simulink model "sl_spmsm"  (R2023b)
settings: Solver=VariableStepAuto  StartTime=0.0  StopTime=10.0  RelTol=1e-3
InitFcn:
  | init
values from neighbouring files (symbols this model uses):
  pa = block.DialogPrm(1).Data    [SPMSM_abc_model.m]    (also in park.m; pwm.m; torque_equation.m; voltage_equation.m)
libraries: slpidlib x1
settings Model: Creator=PC  LastModifiedBy=PC

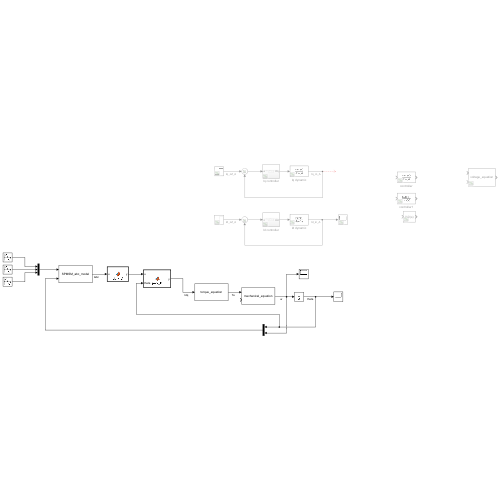
[thumbnail: Simulink's stored preview of the top-level diagram]
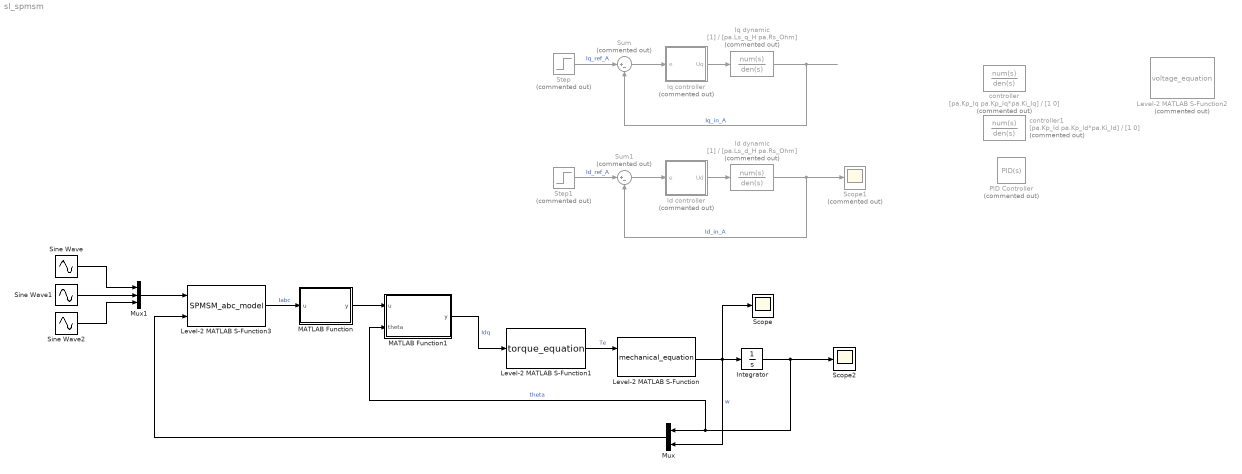
== system sl_spmsm ==
  Id controller : Subsystem  Commented=on
  Id dynamic : TransferFcn  Commented=on  Denominator=[pa.Ls_d_H pa.Rs_Ohm]
  Integrator : Integrator
  Iq controller : Subsystem  Commented=on
  Iq dynamic : TransferFcn  Commented=on  Denominator=[pa.Ls_q_H pa.Rs_Ohm]
  Level-2 MATLAB S-Function : M-S-Function  FunctionName=mechanical_equation  Parameters=pa
  Level-2 MATLAB S-Function1 : M-S-Function  FunctionName=torque_equation  Parameters=pa
  Level-2 MATLAB S-Function2 : M-S-Function  Commented=on  FunctionName=voltage_equation  Parameters=pa
  Level-2 MATLAB S-Function3 : M-S-Function  FunctionName=SPMSM_abc_model  Parameters=pa
  MATLAB Function : MATLAB Function  TreatAsAtomicUnit=on
  MATLAB Function1 : MATLAB Function  TreatAsAtomicUnit=on
  Mux : Mux  Inputs=2
  Mux1 : Mux  Inputs=3
  PID Controller : slpidlib/PID Controller  Commented=on  Controller=PID  Form=Parallel  TimeDomain=Continuous-time  UseExternalTs=off  SampleTime=-1  IntegratorMethod=Forward Euler  FilterMethod=Forward Euler  ControllerParametersSource=internal  P=1  I=1  UseKiTs=off  D=0  N=100  UseFilter=on  TunerSelectOption=Transfer Function Based (PID Tuner App)  InitialConditionSource=internal  InitialConditionForIntegrator=0  InitialConditionForFilter=0  DifferentiatorICPrevScaledInput=0  ExternalReset=none  TrackingMode=off  Kt=1  LimitOutput=off  SatLimitsSource=internal  UpperSaturationLimit=inf  LowerSaturationLimit=-inf  LinearizeAsGain=on  AntiWindupMode=none  Kb=1  LimitIntegrator=off  UpperIntegratorSaturationLimit=inf  LowerIntegratorSaturationLimit=-inf  POutMin=[]  POutMax=[]  IOutMin=[]  IOutMax=[]  DOutMin=[]  DOutMax=[]  NOutMin=[]  NOutMax=[]  SumOutMin=[]  SumOutMax=[]  SaturationOutMin=[]  SaturationOutMax=[]  PParamMin=[]  PParamMax=[]  IParamMin=[]  IParamMax=[]  DParamMin=[]  DParamMax=[]  NParamMin=[]  NParamMax=[]  KbParamMin=[]  KbParamMax=[]  KtParamMin=[]  KtParamMax=[]  KbOutMin=[]  KbOutMax=[]  KtOutMin=[]  KtOutMax=[]  IntegratorOutMin=[]  IntegratorOutMax=[]  FilterOutMin=[]  FilterOutMax=[]  SumI1OutMin=[]  SumI1OutMax=[]  SumI2OutMin=[]  SumI2OutMax=[]  SumI3OutMin=[]  SumI3OutMax=[]  SumI4OutMin=[]  SumI4OutMax=[]  SumDOutMin=[]  SumDOutMax=[]  DifferentiatorOutMin=[]  DifferentiatorOutMax=[]  FilterDiffOutCoefMin=[]  FilterDiffOutCoefMax=[]  ReciprocalOutMin=[]  ReciprocalOutMax=[]  SumDenOutMin=[]  SumDenOutMax=[]  SumNumOutMin=[]  SumNumOutMax=[]  DivideOutMin=[]  DivideOutMax=[]  UdiffTsProdOutMin=[]  UdiffTsProdOutMax=[]  NTsProdOutMin=[]  NTsProdOutMax=[]  UintegralTsProdOutMin=[]  UintegralTsProdOutMax=[]  UngainTsProdOutMin=[]  UngainTsProdOutMax=[]  ClampingZeroOutDataTypeStr=Inherit: Inherit via back propagation  ClampingZeroOutMin=[]  ClampingZeroOutMax=[]  FilterDenConstantOutDataTypeStr=Inherit: Inherit via back propagation  FilterDenConstantOutMin=[]  FilterDenConstantOutMax=[]  PCopyOutDataTypeStr=Inherit: Inherit via back propagation  PCopyOutMin=[]  PCopyOutMax=[]  NCopyOutDataTypeStr=Inherit: Inherit via back propagation  NCopyOutMin=[]  NCopyOutMax=[]  IntegratorContinuousStateAttributes=''  IntegratorStateMustResolveToSignalObject=off  IntegratorRTWStateStorageClass=Auto  FilterContinuousStateAttributes=''  FilterStateMustResolveToSignalObject=off  FilterRTWStateStorageClass=Auto  ParallelPVariant=InternalParameters  IdealPVariant=Disabled  IVariant=InternalParameters  DVariant=InternalParameters  IntegratorVariant=Continuous  SatVariant=Disabled  AWVariant=Passthrough  PCopyVariant=Disabled  TRVariant=Disabled  FdbkBlocksVariant=Forward  IdealPFdbkVariant=Disabled  SatFdbkVariant=Disabled  DerivativeFilterVariant=ContFilter  NVariant=InternalParameters  NCopyVariant=Disabled  FilterICVariant=InternalICsFilter  IntegratorICVariant=InternalICs  ExternalResetVariant=Disabled  TRSumVariant=Passthrough  SumFdbkVariant=Disabled  SumVariant=Sum_PID  TsampFilterVariant=InternalTs  TsampNgainVariant=Passthrough  TsampIntegralVariant=Disabled_SignalSpec  ExternalSaturationOutDataTypeStr=Inherit: Same as second input
  Scope : Scope
  Scope1 : Scope  Commented=on
  Scope2 : Scope
  Sine Wave : Sin  SampleTime=0
  Sine Wave1 : Sin  Phase=-2*pi/3  SampleTime=0
  Sine Wave2 : Sin  Phase=2*pi/3  SampleTime=0
  Step : Step  Commented=on  SampleTime=0
  Step1 : Step  Commented=on  SampleTime=0
  Sum : Sum  Commented=on  Inputs=|+-
  Sum1 : Sum  Commented=on  Inputs=|+-
  controller : TransferFcn  Commented=on  Numerator=[pa.Kp_Iq pa.Kp_Iq*pa.Ki_Iq]  Denominator=[1 0]
  controller1 : TransferFcn  Commented=on  Numerator=[pa.Kp_Id pa.Kp_Id*pa.Ki_Id]  Denominator=[1 0]
  wires:
  Iq dynamic/1 -> Sum/2  "Iq_in_A"
  Id dynamic/1 -> Sum1/2, Scope1/1  "Id_in_A"
  Step/1 -> Sum/1  "Iq_ref_A"
  Id controller/1(Ud) -> Id dynamic/1
  Step1/1 -> Sum1/1  "Id_ref_A"
  Sum/1 -> Iq controller/1(e)
  Iq controller/1(Uq) -> Iq dynamic/1
  Sum1/1 -> Id controller/1(e)
  Level-2 MATLAB S-Function1/1 -> Level-2 MATLAB S-Function/1  "Te"
  Level-2 MATLAB S-Function/1 -> Scope/1, Mux/2, Integrator/1  "w"
  MATLAB Function1/1(y) -> Level-2 MATLAB S-Function1/1  "Idq"
  Integrator/1 -> MATLAB Function1/2(theta), Mux/1, Scope2/1  "theta"
  Mux/1 -> Level-2 MATLAB S-Function3/2
  Level-2 MATLAB S-Function3/1 -> MATLAB Function/1(u)  "Iabc"
  MATLAB Function/1(y) -> MATLAB Function1/1(u)
  Sine Wave/1 -> Mux1/1
  Sine Wave1/1 -> Mux1/2
  Sine Wave2/1 -> Mux1/3
  Mux1/1 -> Level-2 MATLAB S-Function3/1

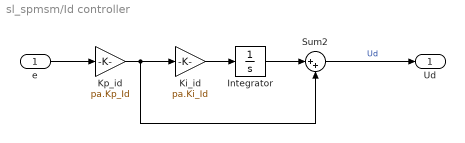
== system sl_spmsm/Id controller ==
  e : Inport
  Integrator : Integrator
  Ki_id : Gain  Gain=pa.Ki_Id
  Kp_id : Gain  Gain=pa.Kp_Id
  Sum2 : Sum  Inputs=|++
  Ud : Outport
  wires:
  Sum2/1 -> Ud/1  "Ud"
  Ki_id/1 -> Integrator/1
  e/1 -> Kp_id/1
  Kp_id/1 -> Ki_id/1, Sum2/2
  Integrator/1 -> Sum2/1

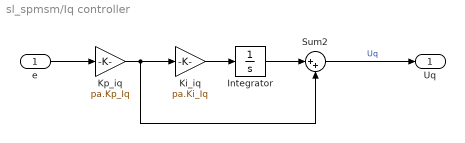
== system sl_spmsm/Iq controller ==
  e : Inport
  Integrator : Integrator
  Ki_iq : Gain  Gain=pa.Ki_Iq
  Kp_iq : Gain  Gain=pa.Kp_Iq
  Sum2 : Sum  Inputs=|++
  Uq : Outport
  wires:
  Integrator/1 -> Sum2/1
  Kp_iq/1 -> Sum2/2, Ki_iq/1
  e/1 -> Kp_iq/1
  Ki_iq/1 -> Integrator/1
  Sum2/1 -> Uq/1  "Uq"

== matlab function sl_spmsm/MATLAB Function ==
  data: u input; y output
function y = clark_tf(u)
clark = 2/3 * [1 -1/2 -1/2;
               0 sqrt(3)/2 -sqrt(3)/2];
y = clark*u;

== matlab function sl_spmsm/MATLAB Function1 ==
  data: u input; y output; theta input
function y = park_tf(u,theta)
park = [cos(theta) sin(theta);
        -sin(theta) cos(theta)];
y = park*u;
